simulink model "Sim_lk"  (R2018b)
settings: Solver=VariableStepAuto  StartTime=0.0  StopTime=0.8  FixedStep=0.001  RelTol=1e-3
values from neighbouring files (symbols this model uses):
  Kb = 18.48e-3    (= 0.01848)    [Lock_key_2018b.m]
  L = 0.231e-3    (= 0.000231)    [Lock_key_2018b.m]
  m = 300e-3    (= 0.3)    [Lock_key_2018b.m]
  R = 3.69    [Lock_key_2018b.m]
undefined symbols (not defined in the file or in its folder): b, Fc, g, Je1, Je2, Ki, rp
settings Model: Creator=Sharan Aakash  LastModifiedBy=Sharan Aakash

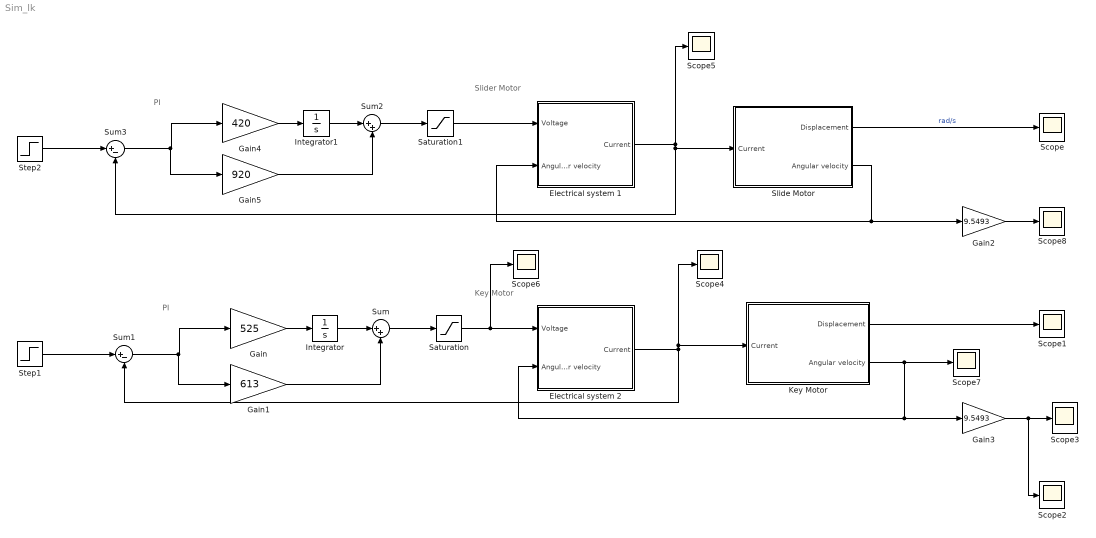
== system Sim_lk ==
  note: PI
  note: Slider Motor
  note: Key Motor
  note: PI
  Electrical system 1 : Subsystem
  Electrical system 2 : Subsystem
  Gain : Gain  Gain=525
  Gain1 : Gain  Gain=613
  Gain2 : Gain  Gain=9.5493
  Gain3 : Gain  Gain=9.5493
  Gain4 : Gain  Gain=420
  Gain5 : Gain  Gain=920
  Integrator : Integrator
  Integrator1 : Integrator
  Key Motor : Subsystem
  Saturation : Saturate  UpperLimit=12
  Saturation1 : Saturate  UpperLimit=12
  Scope{,1..8} (9 alike) : Scope
  Slide Motor : Subsystem
  Step1 : Step  Time=0.05  After=0.818  SampleTime=0
  Step2 : Step  Time=0.05  After=0.818  SampleTime=0
  Sum : Sum  Inputs=|++
  Sum1 : Sum  Inputs=|+-
  Sum2 : Sum  Inputs=|++
  Sum3 : Sum  Inputs=|+-
  wires:
  Slide Motor/2(Angular velocity) -> Electrical system 1/2(Angular velocity), Gain2/1
  Key Motor/1(Displacement) -> Scope1/1
  Slide Motor/1(Displacement) -> Scope/1  "rad/s"
  Gain2/1 -> Scope8/1
  Gain/1 -> Integrator/1
  Saturation1/1 -> Electrical system 1/1(Voltage)
  Saturation/1 -> Scope6/1, Electrical system 2/1(Voltage)
  Sum1/1 -> Gain1/1, Gain/1
  Electrical system 2/1("Current ") -> Scope4/1, Key Motor/1(Current), Sum1/2
  Key Motor/2("Angular velocity ") -> Scope7/1, Gain3/1, Electrical system 2/2(Angular velocity)
  Integrator/1 -> Sum/1
  Gain1/1 -> Sum/2
  Step1/1 -> Sum1/1
  Sum/1 -> Saturation/1
  Gain4/1 -> Integrator1/1
  Step2/1 -> Sum3/1
  Sum2/1 -> Saturation1/1
  Electrical system 1/1("Current ") -> Sum3/2, Slide Motor/1(Current), Scope5/1
  Gain5/1 -> Sum2/2
  Sum3/1 -> Gain5/1, Gain4/1
  Integrator1/1 -> Sum2/1
  Gain3/1 -> Scope2/1, Scope3/1

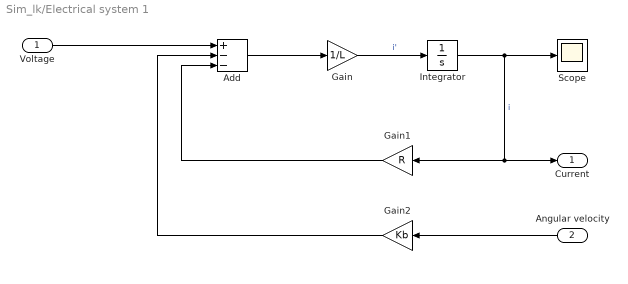
== system Sim_lk/Electrical system 1 ==
  Voltage : Inport
  Angular velocity : Inport  Port=2
  Add : Sum  Inputs=+--
  Gain : Gain  Gain=1/L
  Gain1 : Gain  Gain=R
  Gain2 : Gain  Gain=Kb
  Integrator : Integrator
  Scope : Scope
  "Current " : Outport
  wires:
  Integrator/1 -> Gain1/1, "Current "/1, Scope/1  "i"
  Gain/1 -> Integrator/1  "i'"
  Angular velocity/1 -> Gain2/1
  Add/1 -> Gain/1
  Gain2/1 -> Add/2
  Voltage/1 -> Add/1
  Gain1/1 -> Add/3

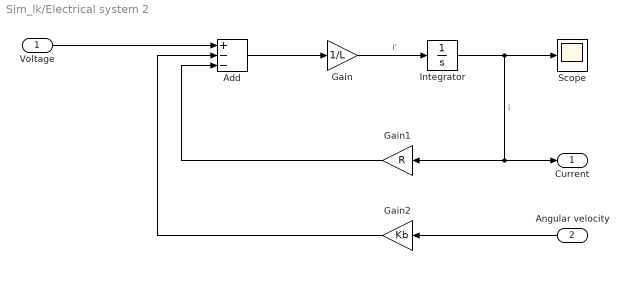
== system Sim_lk/Electrical system 2 ==
  Voltage : Inport
  Angular velocity : Inport  Port=2
  Add : Sum  Inputs=+--
  Gain : Gain  Gain=1/L
  Gain1 : Gain  Gain=R
  Gain2 : Gain  Gain=Kb
  Integrator : Integrator
  Scope : Scope
  "Current " : Outport
  wires:
  Gain1/1 -> Add/3
  Voltage/1 -> Add/1
  Gain2/1 -> Add/2
  Add/1 -> Gain/1
  Angular velocity/1 -> Gain2/1
  Gain/1 -> Integrator/1  "i'"
  Integrator/1 -> Scope/1, "Current "/1, Gain1/1  "i"

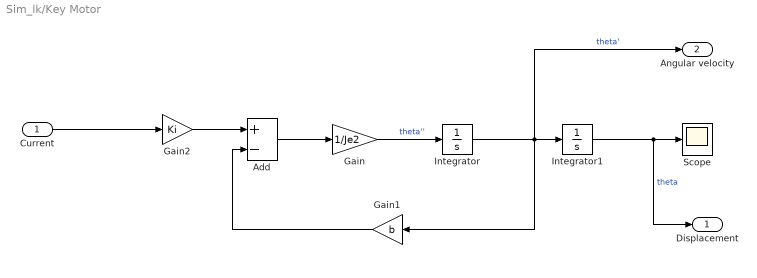
== system Sim_lk/Key Motor ==
  Current : Inport
  Add : Sum  Inputs=+-
  Gain : Gain  Gain=1/Je2
  Gain1 : Gain  Gain=b
  Gain2 : Gain  Gain=Ki
  Integrator : Integrator
  Integrator1 : Integrator
  Scope : Scope
  Displacement : Outport
  "Angular velocity " : Outport  Port=2
  wires:
  Gain2/1 -> Add/1
  Current/1 -> Gain2/1
  Integrator1/1 -> Scope/1, Displacement/1  "theta"
  Gain/1 -> Integrator/1  "theta''"
  Add/1 -> Gain/1
  Gain1/1 -> Add/2
  Integrator/1 -> "Angular velocity "/1, Integrator1/1, Gain1/1  "theta'"

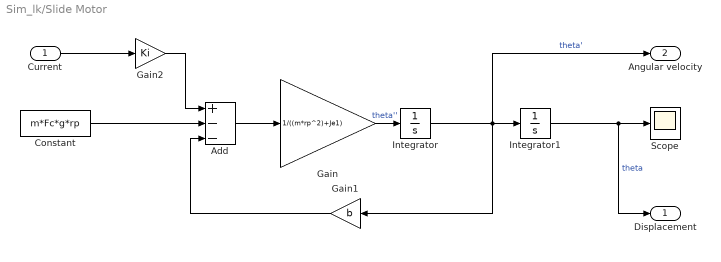
== system Sim_lk/Slide Motor ==
  Current : Inport
  Add : Sum  Inputs=+--
  Constant : Constant  Value=m*Fc*g*rp
  Gain : Gain  Gain=1/((m*rp^2)+Je1)
  Gain1 : Gain  Gain=b
  Gain2 : Gain  Gain=Ki
  Integrator : Integrator
  Integrator1 : Integrator
  Scope : Scope
  Displacement : Outport
  Angular velocity : Outport  Port=2
  wires:
  Integrator/1 -> Angular velocity/1, Gain1/1, Integrator1/1  "theta'"
  Gain1/1 -> Add/3
  Add/1 -> Gain/1
  Gain/1 -> Integrator/1  "theta''"
  Constant/1 -> Add/2
  Integrator1/1 -> Displacement/1, Scope/1  "theta"
  Current/1 -> Gain2/1
  Gain2/1 -> Add/1
